simulink model "Compliance"  (R2021a)
settings: Solver=VariableStepAuto  StartTime=0.0  StopTime=3  RelTol=1e-3
values from neighbouring files (symbols this model uses):
  kd = 2*z*w    [params.m]
  kp = w^2    [params.m]
  x = [    0.4800 ... (first row only)    [params.m]
settings Model: Creator=Sebastiano  LastModifiedBy=antoninoparisi
settings SolverCC: AlgebraicLoopSolver=TrustRegion
settings DebuggingCC: SFMachineParentedDataDiag=warning

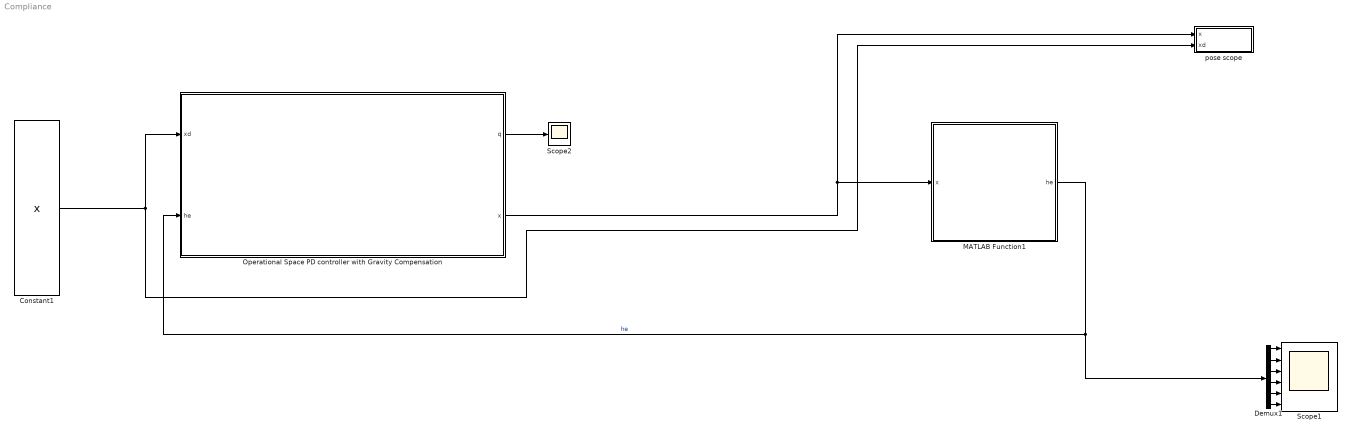
== system Compliance ==
  Constant1 : Constant  Value=x  VectorParams1D=off
  Demux1 : Demux  Outputs=6
  MATLAB Function1 : MATLAB Function  TreatAsAtomicUnit=on
  Operational Space PD controller with Gravity Compensation : Subsystem
  Scope1 : Scope  NumInputPorts=6
  Scope2 : Scope
  pose scope : Subsystem
  wires:
  Constant1/1 -> pose scope/2(xd), Operational Space PD controller with Gravity Compensation/1(xd)
  MATLAB Function1/1(he) -> Operational Space PD controller with Gravity Compensation/2(he), Demux1/1  "he"
  Operational Space PD controller with Gravity Compensation/1(q) -> Scope2/1
  Operational Space PD controller with Gravity Compensation/2(x) -> pose scope/1(x), MATLAB Function1/1(x)
  Demux1/1 -> Scope1/1
  Demux1/6 -> Scope1/6
  Demux1/5 -> Scope1/5
  Demux1/3 -> Scope1/3
  Demux1/2 -> Scope1/2
  Demux1/4 -> Scope1/4

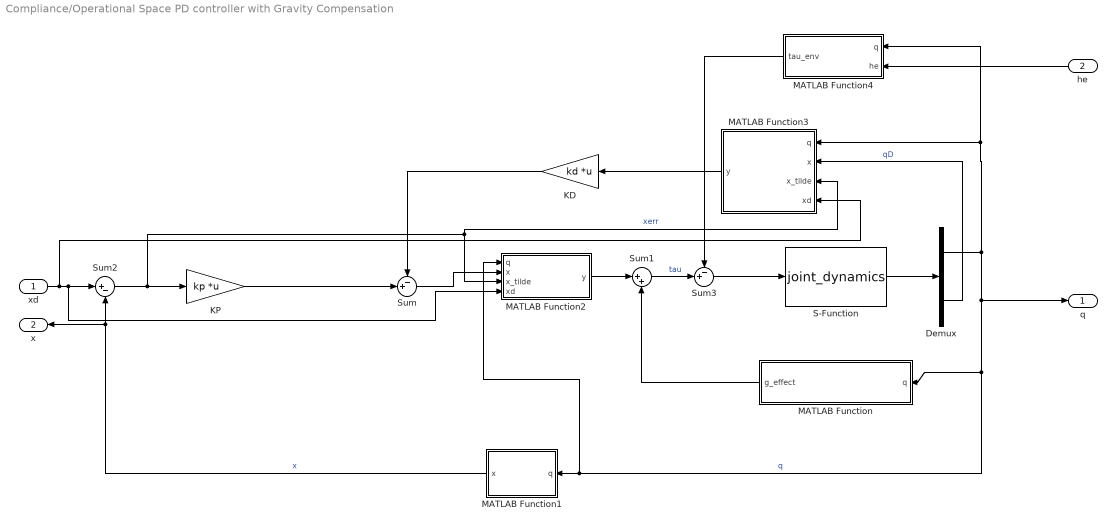
== system Compliance/Operational Space PD controller with Gravity Compensation ==
  xd : Inport
  he : Inport  Port=2
  Demux : Demux  Outputs=[3, 3]
  KD : Gain  Gain=kd  Multiplication=Matrix(K*u) (u vector)
  KP : Gain  Gain=kp  Multiplication=Matrix(K*u) (u vector)
  MATLAB Function : MATLAB Function  TreatAsAtomicUnit=on
  MATLAB Function1 : MATLAB Function  TreatAsAtomicUnit=on
  MATLAB Function2 : MATLAB Function  TreatAsAtomicUnit=on
  MATLAB Function3 : MATLAB Function  TreatAsAtomicUnit=on
  MATLAB Function4 : MATLAB Function  TreatAsAtomicUnit=on
  S-Function : S-Function  FunctionName=joint_dynamics  Parameters=robot  SFunctionDeploymentMode=off  EnableBusSupport=off
  Sum : Sum  Inputs=-+|
  Sum1 : Sum  Inputs=|++
  Sum2 : Sum  Inputs=|+-
  Sum3 : Sum  Inputs=-+|
  q : Outport
  x : Outport  Port=2
  wires:
  MATLAB Function3/1(y) -> KD/1
  Sum/1 -> MATLAB Function2/2(x)
  S-Function/1 -> Demux/1
  KP/1 -> Sum/2
  Sum2/1 -> MATLAB Function2/3(x_tilde), MATLAB Function3/3(x_tilde), KP/1  "xerr"
  Demux/2 -> MATLAB Function3/2(x)  "qD"
  MATLAB Function/1(g_effect) -> Sum1/2
  MATLAB Function1/1(x) -> x/1, Sum2/2  "x"
  Sum3/1 -> S-Function/1
  KD/1 -> Sum/1
  MATLAB Function2/1(y) -> Sum1/1
  Demux/1 -> q/1, MATLAB Function1/1(q), MATLAB Function2/1(q), MATLAB Function/1(q), MATLAB Function4/1(q), MATLAB Function3/1(q)  "q"
  Sum1/1 -> Sum3/2  "tau"
  xd/1 -> MATLAB Function3/4(xd), MATLAB Function2/4(xd), Sum2/1
  MATLAB Function4/1(tau_env) -> Sum3/1
  he/1 -> MATLAB Function4/2(he)

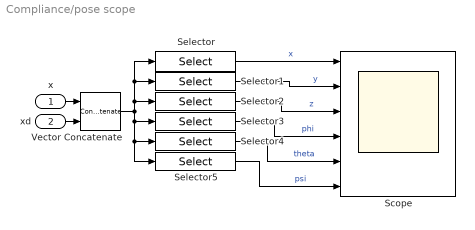
== system Compliance/pose scope ==
  x : Inport
  xd : Inport  Port=2
  Scope : Scope  NumInputPorts=6
  Selector : Selector  NumberOfDimensions=2  InputPortWidth=3  IndexOptions=Index vector (dialog),Select all  Indices=1,7  OutputSizes=6,6
  Selector1 : Selector  NumberOfDimensions=2  InputPortWidth=3  IndexOptions=Index vector (dialog),Select all  Indices=2,7  OutputSizes=6,6
  Selector2 : Selector  NumberOfDimensions=2  InputPortWidth=3  IndexOptions=Index vector (dialog),Select all  Indices=3,7  OutputSizes=6,6
  Selector3 : Selector  NumberOfDimensions=2  InputPortWidth=3  IndexOptions=Index vector (dialog),Select all  Indices=4,7  OutputSizes=6,6
  Selector4 : Selector  NumberOfDimensions=2  InputPortWidth=3  IndexOptions=Index vector (dialog),Select all  Indices=5,7  OutputSizes=6,6
  Selector5 : Selector  NumberOfDimensions=2  InputPortWidth=3  IndexOptions=Index vector (dialog),Select all  Indices=6,7  OutputSizes=6,6
  Vector Concatenate : Concatenate  Mode=Multidimensional array  ConcatenateDimension=2
  wires:
  x/1 -> Vector Concatenate/1
  xd/1 -> Vector Concatenate/2
  Selector1/1 -> Scope/2  "y"
  Selector5/1 -> Scope/6  "psi"
  Selector3/1 -> Scope/4  "phi"
  Selector/1 -> Scope/1  "x"
  Selector4/1 -> Scope/5  "theta"
  Vector Concatenate/1 -> Selector/1, Selector1/1, Selector2/1, Selector5/1, Selector4/1, Selector3/1
  Selector2/1 -> Scope/3  "z"

== matlab function Compliance/MATLAB Function1 ==
  data: x input; he output
function he = environment(x)

% environment params
K = eye(6)*2;    % stiffness
wall = 0.16; % position w.r.t. frame 0 

if x(3) >= wall  
    xe_wall = x;
    xe_wall(3) = wall; % rest position of wall
    % calculate the forces
    dx_ed = x-xe_wall; % manipulator position - env. rest position
    he = K * dx_ed; % spring force by prev displacement for he 
else
    % free motion
    he = zeros(6,1);
end

he = reshape(he,[6 1]);

== matlab function Compliance/Operational Space PD controller with Gravity Compensation/MATLAB Function ==
  data: q input; g_effect output
function g_effect = gravity(q)

g_effect = G_Lagrangian(q);

== matlab function Compliance/Operational Space PD controller with Gravity Compensation/MATLAB Function2 ==
  data: q input; y output size=[3 1]; x input; x_tilde input; xd input
function y = JAT(q, x, x_tilde, xd)


Rd = eul2rotm(xd(4:6)','ZYZ'); % desired frame rm


Phi = x_tilde(4:6);
k   = Phi(1);
t   = Phi(2);



T = [0, -sin(k), cos(k)*sin(t);
     0,  cos(k), sin(k)*sin(t);
     1,       0,        cos(t)];

TA = [eye(3),eye(3)*0;eye(3)*0,T];

J = jacobian(q);

JAd = pinv(TA) * [Rd' zeros(3); zeros(3), Rd']*J;
y = JAd'*x;

== matlab function Compliance/Operational Space PD controller with Gravity Compensation/MATLAB Function3 ==
  data: q input; y output; x input; x_tilde input; xd input
function y = JAT(q, x, x_tilde, xd)


Rd = eul2rotm(xd(4:6)','ZYZ'); % desired ee rotation


Phi = x_tilde(4:6);
k   = Phi(1);
t   = Phi(2);



T = [0, -sin(k), cos(k)*sin(t);
     0,  cos(k), sin(k)*sin(t);
     1,       0,        cos(t)];

TA = [eye(3),eye(3)*0;eye(3)*0,T];

J = jacobian(q);

JA = pinv(TA) * [ Rd' zeros(3); zeros(3), Rd']*J;
y = JA * x;

== matlab function Compliance/Operational Space PD controller with Gravity Compensation/MATLAB Function4 ==
  data: q input; he input; tau_env output
function tau_env = J(q, he)

tau_env = jacobian(q)' * he;

== matlab function Compliance/Operational Space PD controller with Gravity Compensation/MATLAB Function1 ==
  data: q input; x output
function x = K(q)

t1 = q(1);
d1 = q(2);
t2 = q(3);


a1 = 0.15;
a2 = 0.4;
a3 = 0.3;
a4 = 0.16;


% wrt frame 0
K = [[cos(t1)*cos(t2), -cos(t1)*sin(t2), -sin(t1),      a2*cos(t1) + a4*cos(t1)*cos(t2)]
    [        sin(t2),          cos(t2),        0,                 a4*sin(t2) - d1 - a3]
    [cos(t2)*sin(t1), -sin(t1)*sin(t2),  cos(t1), a1 + a2*sin(t1) + a4*cos(t2)*sin(t1)]
    [              0,                0,        0,                                    1]];

pos = K(1:3, 4);
ori = rotm2eul(K(1:3,1:3), 'ZYZ')';

x = [pos; ori];
